simulink model "RI_DI"  (R2013b)
settings: Solver=ode45  StartTime=0.0  StopTime=1  MaxStep=1e-3  RelTol=1e-3
settings Model: Creator=Szalay  LastModifiedBy=Szalay

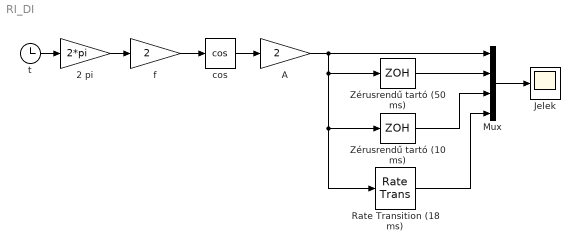
== system RI_DI ==
  2 pi : Gain  Gain=2*pi
  A : Gain  Gain=2
  Jelek : Scope
  Mux : Mux
  Rate Transition (18 ms) : RateTransition  OutPortSampleTime=18e-3
  Zérusrendű tartó (10 ms) : ZeroOrderHold  SampleTime=10e-3
  Zérusrendű tartó (50 ms) : ZeroOrderHold  SampleTime=50e-3
  cos : Trigonometry  Operator=cos
  f : Gain  Gain=2
  t : Clock
  wires:
  t/1 -> 2 pi/1
  2 pi/1 -> f/1
  f/1 -> cos/1
  cos/1 -> A/1
  A/1 -> Mux/1, Zérusrendű tartó (50 ms)/1, Rate Transition (18 ms)/1, Zérusrendű tartó (10 ms)/1
  Zérusrendű tartó (50 ms)/1 -> Mux/2
  Mux/1 -> Jelek/1
  Zérusrendű tartó (10 ms)/1 -> Mux/3
  Rate Transition (18 ms)/1 -> Mux/4
